simulink model "inverter"  (R2016a)
settings: Solver=VariableStepAuto  StartTime=0.0  StopTime=0.02  RelTol=1e-3
libraries: powerlib x15
settings Model: Creator=GADDALA JAYARAJU  LastModifiedBy=GADDALA JAYARAJU

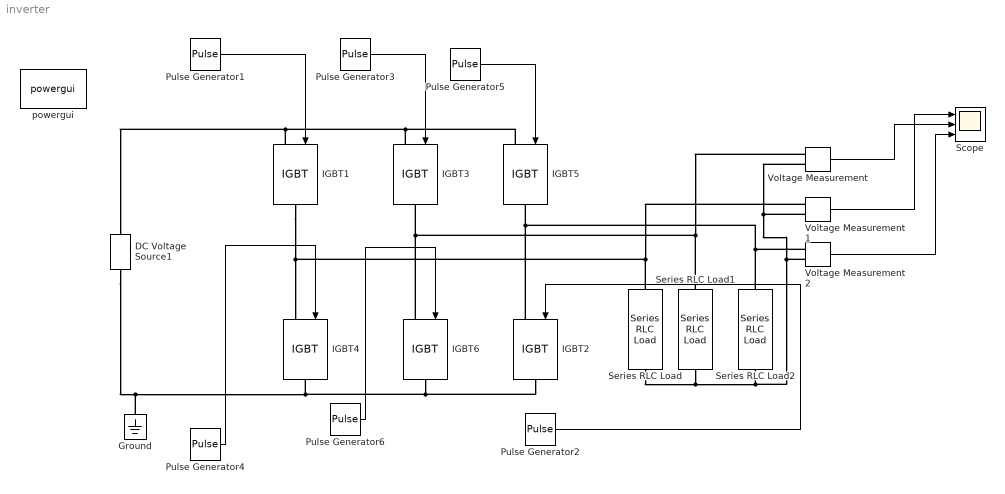
== system inverter ==
  DC Voltage Source1 : powerlib/Electrical Sources/DC Voltage Source  Amplitude=500  Measurements=None
  Ground : powerlib/Elements/Ground  LConnTagsString=a
  IGBT{1..6} (6 alike) : powerlib/Power Electronics/IGBT  Ron=0.001  Lon=0  Vf=1  Tf=1e-6  Tt=2e-6  IC=0  Rs=1e5  Cs=inf  Measurements=off
  Pulse Generator1 : DiscretePulseGenerator  PulseType=Time based  Period=2e-3  PulseWidth=50
  Pulse Generator2 : DiscretePulseGenerator  PulseType=Time based  Period=2e-3  PulseWidth=50  PhaseDelay=(2e-3)*(1/6)
  Pulse Generator3 : DiscretePulseGenerator  PulseType=Time based  Period=2e-3  PulseWidth=50  PhaseDelay=(2e-3)*(2/6)
  Pulse Generator4 : DiscretePulseGenerator  PulseType=Time based  Period=2e-3  PulseWidth=50  PhaseDelay=(2e-3)*(3/6)
  Pulse Generator5 : DiscretePulseGenerator  PulseType=Time based  Period=2e-3  PulseWidth=50  PhaseDelay=(2e-3)*(4/6)
  Pulse Generator6 : DiscretePulseGenerator  PulseType=Time based  Period=2e-3  PulseWidth=50  PhaseDelay=(2e-3)*(5/6)
  Scope : Scope  NumInputPorts=3
  Series RLC Load : powerlib/Elements/Series RLC Load  LConnTagsString=a  RConnTagsString=__new0  NominalVoltage=230  NominalFrequency=50  ActivePower=100  InductivePower=0  CapacitivePower=0  Setx0=off  InitialVoltage=0  SetiL0=off  InitialCurrent=0  Measurements=None  LoadType=constant Z
  Series RLC Load1 : powerlib/Elements/Series RLC Load  LConnTagsString=a  RConnTagsString=__new0  NominalVoltage=230  NominalFrequency=50  ActivePower=100  InductivePower=0  CapacitivePower=0  Setx0=off  InitialVoltage=0  SetiL0=off  InitialCurrent=0  Measurements=None  LoadType=constant Z
  Series RLC Load2 : powerlib/Elements/Series RLC Load  LConnTagsString=a  RConnTagsString=__new0  NominalVoltage=230  NominalFrequency=50  ActivePower=100  InductivePower=0  CapacitivePower=0  Setx0=off  InitialVoltage=0  SetiL0=off  InitialCurrent=0  Measurements=None  LoadType=constant Z
  Voltage Measurement : powerlib/Measurements/Voltage Measurement  PhasorSimulation=off  OutputType=Complex  PSBequivalent=0
  Voltage Measurement1 : powerlib/Measurements/Voltage Measurement  PhasorSimulation=off  OutputType=Complex  PSBequivalent=0
  Voltage Measurement2 : powerlib/Measurements/Voltage Measurement  PhasorSimulation=off  OutputType=Complex  PSBequivalent=0
  powergui : powerlib/powergui  Priority=1  SimulationMode=Discrete  SolverType=Tustin/Backward Euler (TBE)  SampleTime=50e-6  frequency=60  SPID=off  DisableSnubberDevices=off  DisableRonSwitches=off  DisableVfSwitches=off  SwTol=0  DisplayEquations=off  Interpol=off  ExternalGateDelay=off  methode=off  Ts=10  FunctionMessages=off  echomessages=off  HookPort=off  EnableUseOfTLC=off  x0status=blocks  frequencyindice=0  Pbase=100e6  ErrMax=1e-4  Iterations=50  UnitsV=kV  UnitsW=MW  buscounter=0  RestoreLinks=warning  ResistiveCurrentMeasurement=off  Frange=[0:2:500]  Ylog=off  Xlog=on  ShowGrid=off  save=off  variable=ZData  structure=0  ZoomFFT=off  StartTime=0.0  cycles=1  DisplayStyle=1  fundamental=60  FreqAxis=off  MaxFrequency=1000  frequencyindicesteady=1  RmsSteady=1  display=off
  wires:
  Pulse Generator1/1 -> IGBT1/1
  Pulse Generator3/1 -> IGBT3/1
  Pulse Generator5/1 -> IGBT5/1
  Voltage Measurement/1 -> Scope/2
  Voltage Measurement2/1 -> Scope/3
  Voltage Measurement1/1 -> Scope/1
  Pulse Generator4/1 -> IGBT4/1
  Pulse Generator6/1 -> IGBT6/1
  Pulse Generator2/1 -> IGBT2/1
  connections:
  IGBT1/LConn1 -- IGBT5/LConn1 -- IGBT3/LConn1 -- DC Voltage Source1/RConn1
  DC Voltage Source1/LConn1 -- Ground/LConn1 -- IGBT2/RConn1 -- IGBT6/RConn1 -- IGBT4/RConn1
  IGBT1/RConn1 -- Series RLC Load/LConn1 -- Voltage Measurement1/LConn1 -- IGBT4/LConn1
  IGBT6/LConn1 -- Series RLC Load1/LConn1 -- Voltage Measurement/LConn1 -- IGBT3/RConn1
  IGBT2/LConn1 -- Voltage Measurement2/LConn1 -- Series RLC Load2/LConn1 -- IGBT5/RConn1
  Series RLC Load/RConn1 -- Voltage Measurement2/LConn2 -- Voltage Measurement1/LConn2 -- Voltage Measurement/LConn2 -- Series RLC Load2/RConn1 -- Series RLC Load1/RConn1
